simulink model "proj"  (R2015a)
settings: Solver=ode45  StartTime=0.0  StopTime=2.5  RelTol=1e-3
undefined symbols (not defined in the file): D1, Delta, sigbuilder_block
libraries: powerlib x25, powerlib_meascontrol x15, simulink x2, re_lib x1
settings Model: Creator=Lenovo  LastModifiedBy=Lenovo

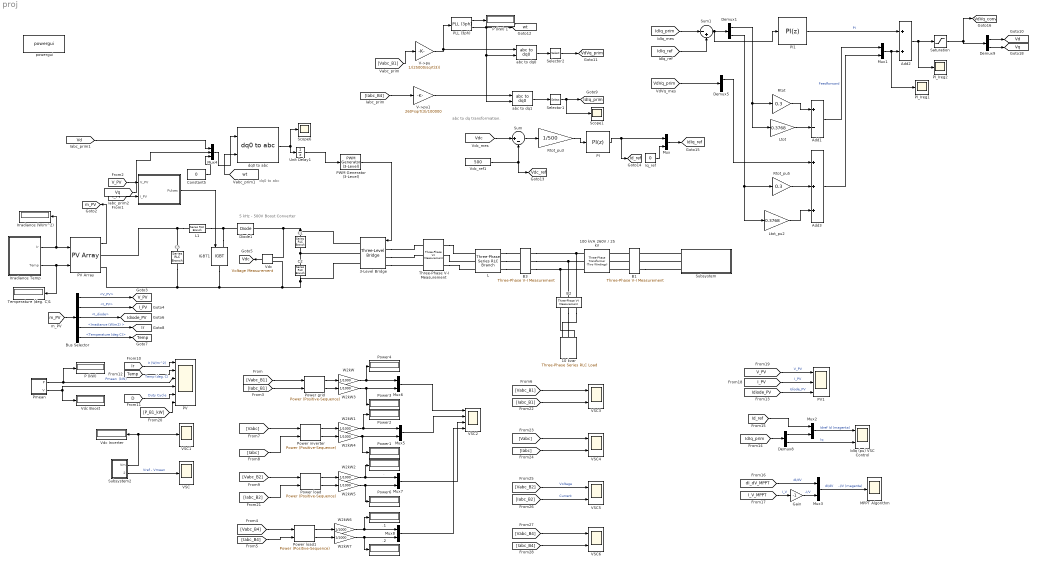
== system proj ==
  note: dq0 to abc
  note: abc to dq transformation.
  note: 5 kHz - 500V
      | Boost Converter
  " " : Subsystem  mask(Boost Control - MPPT){fc=5000, T_MPPT=200e-6, Dinit=0.5}
      mask prompts: fc "PWM switching frequency (Hz)"; T_MPPT "Time window used by MPPT control (s)"; Dinit "Initial value of duty cycle"
  "                                                                                                                                                           ." : Display
      settings: Format=bank  Decimation=2000
  "                                                                                                                                                           .1" : Display
      settings: Format=bank  Decimation=2000
  "                                                                                                                                                           .2" : Display
      settings: Format=bank  Decimation=2000
  10 kvar : powerlib/Elements/Three-Phase Series RLC Load  LConnTagsString=A|B|C  Configuration=Y (grounded)  NominalVoltage=240  NominalFrequency=60  ActivePower=50e3  InductivePower=0  CapacitivePower=0  Measurements=None  LoadType=constant Z
  100 kVA 260V / 25 kV : powerlib/Elements/Three-Phase Transformer (Two Windings)  Winding1Connection=Yg  Winding2Connection=Delta (D1)  CoreType=Three single-phase transformers  SetSaturation=off  Hysteresis=off  DataFile='hysteresis'  SetInitialFlux=off  Measurements=None  UNITS=pu  NominalPower=[100e3 , 60 ]  Winding1=[25000 0.001 0.03]  Winding2=[260 0.001 0.029999]  Rm=500  Lm=500  L0=0.5  Saturation=[0 0;0.0024 1.2;1 1.52]  InitialFluxes=[0.79999 -0.79999 0.7]  MoreParameters=off  BreakLoop=off  DataType=off  TransfoNumber=0
  3-Level Bridge : powerlib/Power Electronics/Three-Level Bridge  Arms=3  SnubberResistance=1e6  SbubberCapacitance=inf  Device=IGBT / Diodes  Ron=0.2e-3  ForwardVoltages="[  0  0 ]"  Measurements=None
  Add1 : Sum  Inputs=+-
  Add2 : Sum
  Add3 : Sum  Inputs=+++
  B1 : powerlib/Measurements/Three-Phase V-I Measurement  VoltageMeasurement=phase-to-ground  SetLabelV=on  LabelV=Vabc_B1  Vpu=off  VpuLL=off  CurrentMeasurement=yes  SetLabelI=on  LabelI=Iabc_B1  Ipu=off  Pbase=100e6  Vbase=500e3  OutputType=Magnitude  PhasorSimulation=off  PSBequivalent=0
  B2 : powerlib/Measurements/Three-Phase V-I Measurement  VoltageMeasurement=phase-to-ground  SetLabelV=on  LabelV=Vabc_B2  Vpu=off  VpuLL=off  CurrentMeasurement=yes  SetLabelI=on  LabelI=Iabc_B2  Ipu=off  Pbase=100e6  Vbase=500e3  OutputType=Magnitude  PhasorSimulation=off  PSBequivalent=0
  B3 : powerlib/Measurements/Three-Phase V-I Measurement  VoltageMeasurement=phase-to-ground  SetLabelV=on  LabelV=Vabc_B4  Vpu=off  VpuLL=off  CurrentMeasurement=yes  SetLabelI=on  LabelI=Iabc_B4  Ipu=off  Pbase=100e6  Vbase=500e3  OutputType=Magnitude  PhasorSimulation=off  PSBequivalent=0
  Bus Selector : BusSelector  OutputSignals=V_PV,I_PV,I_diode,Irradiance (W/m2) ,Temperature (deg C)
  C1 : powerlib/Elements/Series RLC Branch  LConnTagsString=__new0  RConnTagsString=__new0  BranchType=C  Resistance=1.0  Inductance=1.0  SetiL0=off  InitialCurrent=0  Capacitance=12000e-06  Setx0=off  InitialVoltage=0  Measurements=None
  C2 : powerlib/Elements/Series RLC Branch  LConnTagsString=__new0  RConnTagsString=__new0  BranchType=C  Resistance=1.0  Inductance=1.0  SetiL0=off  InitialCurrent=0  Capacitance=12000e-06  Setx0=off  InitialVoltage=0  Measurements=None
  C3 : powerlib/Elements/Series RLC Branch  LConnTagsString=__new0  RConnTagsString=__new0  BranchType=C  Resistance=1.0  Inductance=1.0  SetiL0=off  InitialCurrent=0  Capacitance=100e-6  Setx0=off  InitialVoltage=0  Measurements=Branch voltage
  Constant5 : Constant  Value=0
  Demux{1,5,8..9} (4 alike) : Demux  Outputs=2
  Diode1 : powerlib/Power Electronics/Diode  Ron=1e-4  Lon=0  Vf=0  IC=0  UseSnubber=off  Rs=inf  Cs=inf  Measurements=off
  Gain : Gain  Gain=-1
  IGBT1 : powerlib/Power Electronics/IGBT  Ron=0.001  Lon=0  Vf=0  Tf=0  Tt=0  IC=0  Rs=1e5  Cs=inf  Measurements=off
  IdIq (pu) VSC Control : Scope  NumInputPorts=2
      settings: TimeRange=2  YMin=-5~-5  YMax=5~5  SaveName=ScopeData8  Decimation=100
  Iq_ref : Constant  Value=0
  Irradiance (W/m^2) : Display
      settings: Format=bank  Decimation=1000
  Irradiance Temp : Subsystem  Tag=STV Subsys  LoadFcn=sigbuilder_block('load');  StartFcn=sigbuilder_block('start');  StopFcn=sigbuilder_block('stop');  ClipboardFcn=sigbuilder_block('clipboard');  mask(Sigbuilder block){}
      mask help: Sigbuilder GUI
      mask init:
      | if ~strcmp(get_param(bdroot(gcbh),'SimulationStatus'),'stopped') tuvar = sigbuilder_block('maskInit'); end
      settings: CopyFcn=sigbuilder_block('copy');  DeleteFcn=sigbuilder_block('delete');  ModelCloseFcn=sigbuilder_block('modelClose');  PreSaveFcn=sigbuilder_block('preSave');  PauseFcn=sigbuilder_block('pause')  ContinueFcn=sigbuilder_block('continue')  NameChangeFcn=sigbuilder_block('namechange');  OpenFcn=sigbuilder_block('open',[216.75 153.75 550.5 395.25 ]);  CloseFcn=sigbuilder_block('close');
      mask Display: plot(0,0,100,100,[10,10,40,40,10],[80,20,20,80,80],[40,10],[50,50], [40,27,10],[65,72,56],[40,25,25,10],[28,28,43,43]);
  L : powerlib/Elements/Three-Phase Series RLC Branch  LConnTagsString=A|B|C  RConnTagsString=A|B|C  BranchType=RL  Resistance=0.3  Inductance=1e-3  Capacitance=inf  Measurements=None
  L1 : powerlib/Elements/Series RLC Branch  LConnTagsString=__new0  RConnTagsString=__new0  BranchType=RL  Resistance=0.005  Inductance=5e-3  SetiL0=off  InitialCurrent=0  Capacitance=1e-6  Setx0=off  InitialVoltage=0  Measurements=None
  Ltot : Gain  Gain=0.3768  SaturateOnIntegerOverflow=on  OutDataTypeStr=Inherit: Same as input  ParamDataTypeStr=Inherit: Same as input
  Ltot_pu2 : Gain  Gain=0.3768  SaturateOnIntegerOverflow=on  OutDataTypeStr=Inherit: Same as input  ParamDataTypeStr=Inherit: Same as input
  MPPT Algorithm : Scope
      settings: TimeRange=2  SaveName=ScopeData9  Decimation=100
  Mux{,1..3,5..8} (8 alike) : Mux  Inputs=2
  Mux4 : Mux  Inputs=3
  "P (kW) " : Display
      settings: Format=bank  Decimation=2000
  P (kW) 1 : Display
      settings: Format=bank  Decimation=2000
  PI : simulink/Continuous/PID Controller  Controller=PI  TimeDomain=Discrete-time  SampleTime=1e-06  IntegratorMethod=Trapezoidal  FilterMethod=Forward Euler  Form=Parallel  UseFilter=on  ControllerParametersSource=internal  P=7  I=800  D=0  N=100  InitialConditionSource=internal  InitialConditionForIntegrator=0  InitialConditionForFilter=0  ExternalReset=none  LimitOutput=on  UpperSaturationLimit=1.5  LowerSaturationLimit=-1.5  LinearizeAsGain=off  AntiWindupMode=none  Kb=1  TrackingMode=off  Kt=1  PParamMin=[]  PParamMax=[]  IParamMin=[]  IParamMax=[]  DParamMin=[]  DParamMax=[]  NParamMin=[]  NParamMax=[]  KbParamMin=[]  KbParamMax=[]  KtParamMin=[]  KtParamMax=[]  POutMin=[]  POutMax=[]  IOutMin=[]  IOutMax=[]  DOutMin=[]  DOutMax=[]  NOutMin=[]  NOutMax=[]  KbOutMin=[]  KbOutMax=[]  KtOutMin=[]  KtOutMax=[]  IntegratorOutMin=[]  IntegratorOutMax=[]  FilterOutMin=[]  FilterOutMax=[]  SumOutMin=[]  SumOutMax=[]  SumI1OutMin=[]  SumI1OutMax=[]  SumI2OutMin=[]  SumI2OutMax=[]  SumI3OutMin=[]  SumI3OutMax=[]  SumDOutMin=[]  SumDOutMax=[]  SaturationOutMin=[]  SaturationOutMax=[]  IntegratorContinuousStateAttributes=''  IntegratorStateMustResolveToSignalObject=off  IntegratorRTWStateStorageClass=Auto  FilterContinuousStateAttributes=''  FilterStateMustResolveToSignalObject=off  FilterRTWStateStorageClass=Auto  DifferentiatorICPrevScaledInput=0  DifferentiatorOutMin=[]  DifferentiatorOutMax=[]
  PI1 : simulink/Continuous/PID Controller  Controller=PI  TimeDomain=Discrete-time  SampleTime=1e-06  IntegratorMethod=Forward Euler  FilterMethod=Forward Euler  Form=Parallel  UseFilter=on  ControllerParametersSource=internal  P=0.3  I=20  D=0  N=100  InitialConditionSource=internal  InitialConditionForIntegrator=0  InitialConditionForFilter=0  ExternalReset=none  LimitOutput=on  UpperSaturationLimit=2  LowerSaturationLimit=-2  LinearizeAsGain=off  AntiWindupMode=none  Kb=1  TrackingMode=off  Kt=1  PParamMin=[]  PParamMax=[]  IParamMin=[]  IParamMax=[]  DParamMin=[]  DParamMax=[]  NParamMin=[]  NParamMax=[]  KbParamMin=[]  KbParamMax=[]  KtParamMin=[]  KtParamMax=[]  POutMin=[]  POutMax=[]  IOutMin=[]  IOutMax=[]  DOutMin=[]  DOutMax=[]  NOutMin=[]  NOutMax=[]  KbOutMin=[]  KbOutMax=[]  KtOutMin=[]  KtOutMax=[]  IntegratorOutMin=[]  IntegratorOutMax=[]  FilterOutMin=[]  FilterOutMax=[]  SumOutMin=[]  SumOutMax=[]  SumI1OutMin=[]  SumI1OutMax=[]  SumI2OutMin=[]  SumI2OutMax=[]  SumI3OutMin=[]  SumI3OutMax=[]  SumDOutMin=[]  SumDOutMax=[]  SaturationOutMin=[]  SaturationOutMax=[]  IntegratorContinuousStateAttributes=''  IntegratorStateMustResolveToSignalObject=off  IntegratorRTWStateStorageClass=Auto  FilterContinuousStateAttributes=''  FilterStateMustResolveToSignalObject=off  FilterRTWStateStorageClass=Auto  DifferentiatorICPrevScaledInput=0  DifferentiatorOutMin=[]  DifferentiatorOutMax=[]
  PI_Ireg1 : Scope
      settings: SaveName=ScopeData5
  PI_Ireg2 : Scope
      settings: SaveName=ScopeData13
  PLL (3ph) : powerlib_meascontrol/PLL/PLL (3ph)  Fmin=45  Par_Init="[-0.57  60]"  ParK=[180, 3200, 1]  TcD=1e-4  MaxRateChangeFreq=12  FilterCutOffFreq=25  Ts=1e-06  AGC=on
  PV : Scope  NumInputPorts=6
      settings: TimeRange=2.5  YMin=200~25~0~0~0.44~-5  YMax=1000~50~150~400~0.52~5  SaveName=ScopeData7  Decimation=100
  PV Array : re_lib/Solar/PV Array  Npar=66  Nser=5  PlotType=array @ 1000 W/m2 & specified temperatures  S_vec="[ 1000  250 ]"  Temp_C_vec="[0 25 50  ]"  ModuleName=SunPower SPR-305E-WHT-D  PlotWhenSelected=off  Pm=305.226  Ncell=96  Voc=64.2  Isc=5.96  Vm=54.7  Im=5.58  beta_Voc_pc=-0.27269  alpha_Isc_pc=0.061745  beta_Voc=-0.17507  alpha_Isc=0.00368  IL=6.0092  I0=6.3014e-12  nI=0.94504  Rsh=269.5934  Rs=0.37152  BAL=on  Tc=Tc  Tfilter=5e-5
  PV1 : Scope  NumInputPorts=3
      settings: TimeRange=2  YMin=-5~-5~-5  YMax=5~5~5  SaveName=ScopeData10  Decimation=100
  PWM Generator (3-Level) : powerlib_meascontrol/Pulse & Signal Generators/PWM Generator (3-Level)  ModulatorType=Three-phase bridge (12 pulses)  ModulatorMode=Unsynchronized  nF=27  Fc=33*60  ModulatingSignals=off  m=0.8  Freq=60  Phase=0  Ts=1e-06
  Pmean : Subsystem
  Power grid : powerlib_meascontrol/Measurements/Power (Positive-Sequence)  Freq=60  Vinit=[0, 0]  Iinit=[0, 0]  Ts=1e-06
  Power inverter : powerlib_meascontrol/Measurements/Power (Positive-Sequence)  Freq=60  Vinit=[0, 0]  Iinit=[0, 0]  Ts=1e-06
  Power load : powerlib_meascontrol/Measurements/Power (Positive-Sequence)  Freq=60  Vinit=[0, 0]  Iinit=[0, 0]  Ts=1e-06
  Power load1 : powerlib_meascontrol/Measurements/Power (Positive-Sequence)  Freq=60  Vinit=[0, 0]  Iinit=[0, 0]  Ts=1e-06
  Power{1..4,6} (5 alike) : Display
      settings: Format=bank  Decimation=2000
  Rtot : Gain  Gain=0.3  SaturateOnIntegerOverflow=on  OutDataTypeStr=Inherit: Same as input  ParamDataTypeStr=Inherit: Same as input
  Rtot_pu3 : Gain  Gain=1/500  SaturateOnIntegerOverflow=on  OutDataTypeStr=Inherit: Same as input  ParamDataTypeStr=Inherit: Same as input
  Rtot_pu5 : Gain  Gain=0.3  SaturateOnIntegerOverflow=on  OutDataTypeStr=Inherit: Same as input  ParamDataTypeStr=Inherit: Same as input
  Saturation : Saturate  UpperLimit=2  LowerLimit=-2
  Scope1 : Scope
      settings: YMin=-0.09  YMax=0.06
  Scope6 : Scope
      settings: SaveName=ScopeData14
  Selector1 : Selector  InputPortWidth=3  Indices=[1 2]
  Selector2 : Selector  InputPortWidth=3  Indices=[1 2]
  Subsystem : Subsystem
  Subsystem2 : Subsystem
  Sum : Sum  Inputs=|+-
  Sum1 : Sum  Inputs=|-+
  Temperature (deg. C)1 : Display
      settings: Format=bank  Decimation=1000
  Three-Phase V-I Measurement : powerlib/Measurements/Three-Phase V-I Measurement  VoltageMeasurement=phase-to-ground  SetLabelV=on  LabelV=Vabc  Vpu=off  VpuLL=off  CurrentMeasurement=yes  SetLabelI=on  LabelI=Iabc  Ipu=off  Pbase=100e6  Vbase=500e3  OutputType=Complex  PhasorSimulation=off  PSBequivalent=0
  Unit Delay1 : UnitDelay  SampleTime=1e-06
  V->pu : Gain  Gain=1/(25000/sqrt(3))  SaturateOnIntegerOverflow=on  OutDataTypeStr=Inherit: Same as input  ParamDataTypeStr=Inherit: Same as input
  V->pu1 : Gain  Gain=260*sqrt(3)/100000  SaturateOnIntegerOverflow=on  OutDataTypeStr=Inherit: Same as input  ParamDataTypeStr=Inherit: Same as input
  VSC : Scope
      settings: TimeRange=2.5  SaveName=ScopeData6  Decimation=100
  VSC1 : Scope
      settings: TimeRange=2.5  YMin=499.92  YMax=500.08  SaveName=ScopeData11  Decimation=100
  VSC2 : Scope  NumInputPorts=4
      settings: TimeRange=2.5  YMin=-350~-275~-5~-5  YMax=350~275~5~5  Decimation=100
  VSC{3..6} (4 alike) : Scope  NumInputPorts=2
      VSC3 settings: TimeRange=2.5  YMin=-350~-275  YMax=350~275  SaveName=ScopeData2  Decimation=100
      VSC4 settings: TimeRange=2.5  YMin=-350~-275  YMax=350~275  SaveName=ScopeData3  Decimation=100
      VSC5 settings: TickLabels=on  ShowLegends=on  TimeRange=2.5  YMin=-350~-275  YMax=350~275  SaveName=ScopeData4  Decimation=100
      VSC6 settings: TimeRange=2.5  YMin=-350~-275  YMax=350~275  SaveName=ScopeData12  Decimation=100
  "Vdc " : powerlib/Measurements/Voltage Measurement  Tag=PoWeRsYsTeMmEaSuReMeNt  PhasorSimulation=off  OutputType=Magnitude  PSBequivalent=0
  Vdc Boost : Display
      settings: Format=bank  Decimation=2000
  Vdc Inverter : Display
      settings: Format=bank  Decimation=2000
  Vdc_ref1 : Constant  Value=500
  W2kW{,1..7} (8 alike) : Gain  Gain=1/1000
  abc to dq0 : powerlib_meascontrol/Transformations/abc to dq0  Alignment=90 degrees behind phase A axis
  abc to dq1 : powerlib_meascontrol/Transformations/abc to dq0  Alignment=90 degrees behind phase A axis
  dq0 to abc : powerlib_meascontrol/Transformations/dq0 to abc  Alignment=90 degrees behind phase A axis
  powergui : powerlib/powergui  Priority=1  SimulationMode=Discrete  SolverType=Tustin/Backward Euler (TBE)  SampleTime=1e-06  frequency=60  SPID=off  DisableSnubberDevices=off  DisableRonSwitches=off  DisableVfSwitches=off  SwTol=0  DisplayEquations=off  Interpol=off  methode=off  Ts=0  FunctionMessages=off  echomessages=off  HookPort=off  EnableUseOfTLC=off  x0status=blocks  frequencyindice=0  Pbase=100e6  ErrMax=1e-4  Iterations=50  UnitsV=kV  UnitsW=MW  buscounter=0  RestoreLinks=warning  ResistiveCurrentMeasurement=off  Frange=[0:2:500]  Ylog=off  Xlog=on  ShowGrid=off  save=off  variable=ZData  structure=ScopeData3  ZoomFFT=off  StartTime=0.1  cycles=20  DisplayStyle=1  fundamental=60  FreqAxis=off  MaxFrequency=1000  frequencyindicesteady=1  RmsSteady=1  display=off
  tag scope: I_PV=global, IdIq_prim=global, IdIq_ref=global, Id_ref=global, Idiode_PV=global, Ir=global, Temp=global, V_PV=global, Vd=global, VdVq_conv=global, VdVq_prim=global, Vdc=global, Vdc_ref=global, Vq=global, m_PV=global, wt=global
  wires:
  PV Array/1 -> [m_PV]
  [m_PV] -> Bus Selector/1
  Bus Selector/4 -> [Ir]  "<Irradiance (W/m2) >"
  Bus Selector/5 -> [Temp]  "<Temperature (deg C)>"
  Bus Selector/1 -> [V_PV]  "<V_PV>"
  Bus Selector/2 -> [I_PV]  "<I_PV>"
  Bus Selector/3 -> [Idiode_PV]  "<I_diode>"
  "Vdc "/1 -> [Vdc]
  [I_PV] -> " "/2(I_PV)
  [V_PV] -> " "/1(V_PV)
  [Vabc_B1] -> Power grid/1
  [Iabc_B1] -> Power grid/2
  Power grid/2 -> W2kW3/1
  Power grid/1 -> W2kW/1
  V->pu1/1 -> abc to dq1/1
  V->pu/1 -> PLL (3ph)/1, abc to dq0/1
  abc to dq1/1 -> Selector1/1
  [Vabc_B1] -> V->pu/1
  [Iabc_B4] -> V->pu1/1
  abc to dq0/1 -> Selector2/1
  Selector2/1 -> [VdVq_prim]
  Selector1/1 -> Scope1/1, [IdIq_prim]
  PLL (3ph)/2 -> [wt], abc to dq1/2, abc to dq0/2
  PLL (3ph)/1 -> P (kW) 1/1
  Sum/1 -> Rtot_pu3/1
  [Vdc] -> Sum/1
  Vdc_ref1/1 -> Sum/2, [Vdc_ref]
  Rtot_pu3/1 -> PI/1
  PI/1 -> Mux/1, [Id_ref]
  Iq_ref/1 -> Mux/2
  Mux/1 -> [IdIq_ref]
  Mux1/1 -> PI_Ireg1/1, Add2/2
  PI1/1 -> Add2/1  "PI"
  [IdIq_ref] -> Sum1/2
  [IdIq_prim] -> Sum1/1
  Add2/1 -> PI_Ireg2/1, Saturation/1
  Saturation/1 -> [VdVq_conv], Demux9/1
  [VdVq_prim] -> Demux5/1
  Demux1/1 -> Ltot/1, Rtot/1
  Ltot/1 -> Add1/2
  Demux1/2 -> Rtot_pu5/1, Ltot_pu2/1
  Rtot_pu5/1 -> Add3/2
  Ltot_pu2/1 -> Add3/3
  Add1/1 -> Mux1/1  "Feedforward"
  Add3/1 -> Mux1/2
  Subsystem2/2(VrVm) -> VSC/1  "Vref - Vmean"
  Subsystem2/1(Vm) -> Vdc Inverter/1, VSC1/1
  Pmean/1(P) -> PV/3, "P (kW) "/1  "Pmean  (kW)"
  [D] -> PV/5  "Duty Cycle"
  [Temp] -> PV/2  "Temp (deg. C)"
  [Ir] -> PV/1  "Ir (W/m^2)"
  PWM Generator (3-Level)/1 -> 3-Level Bridge/1
  " "/1(Pulses) -> IGBT1/1
  [I_V_MPPT] -> Gain/1  "I_V"
  [IdIq_prim] -> Demux8/1
  [Id_ref] -> Mux2/1
  Demux8/1 -> Mux2/2
  Mux2/1 -> IdIq (pu) VSC Control/1  "Idref Id (magenta)"
  Demux8/2 -> IdIq (pu) VSC Control/2  "Iq"
  [V_PV] -> PV1/1  "V_PV"
  [I_PV] -> PV1/2  "I_PV"
  [Idiode_PV] -> PV1/3  "Idiode_PV"
  [dI_dV_MPPT] -> Mux3/1  "dI/dV"
  Gain/1 -> Mux3/2  "-I/V"
  Mux3/1 -> MPPT Algorithm/1  "dI/dV     -I/V (magenta)"
  Demux9/1 -> [Vd]
  Demux9/2 -> [Vq]
  [Vq] -> Mux4/2
  [Vd] -> Mux4/1
  Constant5/1 -> Mux4/3
  Mux4/1 -> dq0 to abc/1
  [wt] -> dq0 to abc/2
  dq0 to abc/1 -> Unit Delay1/1, Scope6/1
  Unit Delay1/1 -> PWM Generator (3-Level)/1
  [P_B1_kW] -> PV/6
  [Vabc] -> Power inverter/1
  [Iabc] -> Power inverter/2
  Power inverter/1 -> W2kW1/1
  W2kW1/1 -> Power2/1, Mux5/1
  [Vabc_B2] -> Power load/1
  [Iabc_B2] -> Power load/2
  Power load/1 -> W2kW2/1
  W2kW2/1 -> "                                                                                                                                                           ."/1, Mux7/1
  W2kW3/1 -> Power3/1, Mux6/2
  Power inverter/2 -> W2kW4/1
  W2kW4/1 -> Power1/1, Mux5/2
  [Vabc_B4] -> Power load1/1
  [Iabc_B4] -> Power load1/2
  Sum1/1 -> PI1/1, Demux1/1
  Demux5/1 -> Add3/1
  Rtot/1 -> Add1/1
  Pmean/2(V) -> Vdc Boost/1, PV/4
  W2kW/1 -> Power4/1, Mux6/1
  Power load/2 -> W2kW5/1
  W2kW5/1 -> Power6/1, Mux7/2
  Mux6/1 -> VSC2/1
  Mux5/1 -> VSC2/2
  Mux7/1 -> VSC2/3
  Power load1/1 -> W2kW6/1
  Power load1/2 -> W2kW7/1
  W2kW6/1 -> "                                                                                                                                                           .1"/1, Mux8/1
  W2kW7/1 -> "                                                                                                                                                           .2"/1, Mux8/2
  Mux8/1 -> VSC2/4
  [Vabc_B1] -> VSC3/1
  [Iabc_B1] -> VSC3/2
  [Vabc] -> VSC4/1
  [Iabc] -> VSC4/2
  [Vabc_B2] -> VSC5/1  "Voltage"
  [Iabc_B2] -> VSC5/2  "Current"
  [Vabc_B4] -> VSC6/1
  [Iabc_B4] -> VSC6/2
  Irradiance Temp/1(Ir) -> PV Array/1, Irradiance (W/m^2)/1
  Irradiance Temp/2(Temp) -> PV Array/2, Temperature (deg. C)1/1
  connections:
  Diode1/RConn1 -- "Vdc "/LConn1 -- 3-Level Bridge/RConn1 -- C1/LConn1
  IGBT1/LConn1 -- L1/RConn1 -- Diode1/LConn1
  IGBT1/RConn1 -- PV Array/RConn2 -- C3/RConn1 -- 3-Level Bridge/RConn3 -- C2/RConn1 -- "Vdc "/LConn2
  C2/LConn1 -- 3-Level Bridge/RConn2 -- C1/RConn1
  L1/LConn1 -- PV Array/RConn1 -- C3/LConn1
  B2/LConn2 -- B3/RConn2 -- 100 kVA 260V / 25 kV/RConn2
  3-Level Bridge/LConn1 -- Three-Phase V-I Measurement/LConn1
  3-Level Bridge/LConn2 -- Three-Phase V-I Measurement/LConn2
  3-Level Bridge/LConn3 -- Three-Phase V-I Measurement/LConn3
  Three-Phase V-I Measurement/RConn1 -- L/LConn1
  Three-Phase V-I Measurement/RConn2 -- L/LConn2
  Three-Phase V-I Measurement/RConn3 -- L/LConn3
  B1/LConn1 -- 100 kVA 260V / 25 kV/LConn1
  B1/LConn2 -- 100 kVA 260V / 25 kV/LConn2
  B1/LConn3 -- 100 kVA 260V / 25 kV/LConn3
  B2/LConn1 -- 100 kVA 260V / 25 kV/RConn1 -- B3/RConn1
  B2/LConn3 -- 100 kVA 260V / 25 kV/RConn3 -- B3/RConn3
  Subsystem/LConn1 -- B1/RConn1
  Subsystem/LConn2 -- B1/RConn2
  B1/RConn3 -- Subsystem/LConn3
  B2/RConn1 -- 10 kvar/LConn1
  B2/RConn2 -- 10 kvar/LConn2
  10 kvar/LConn3 -- B2/RConn3
  L/RConn1 -- B3/LConn1
  L/RConn2 -- B3/LConn2
  L/RConn3 -- B3/LConn3

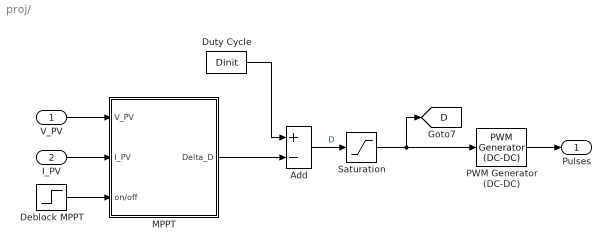
== system proj/  ==
  V_PV : Inport
  I_PV : Inport  Port=2
  Add : Sum  Inputs=+-
  Deblock MPPT : Step  Time=0.1  SampleTime=0
  Duty Cycle : Constant  Value=Dinit
  MPPT : Subsystem
  PWM Generator (DC-DC) : powerlib_meascontrol/Pulse & Signal Generators/PWM Generator (DC-DC)  Fsw=fc  Ts=1e-06
  Saturation : Saturate  UpperLimit=1  LowerLimit=0
  Pulses : Outport
  tag scope: D=global
  wires:
  V_PV/1 -> MPPT/1(V_PV)
  I_PV/1 -> MPPT/2(I_PV)
  PWM Generator (DC-DC)/1 -> Pulses/1
  Deblock MPPT/1 -> MPPT/3(on/off)
  Saturation/1 -> PWM Generator (DC-DC)/1, [D]
  Add/1 -> Saturation/1  "D"
  MPPT/1(Delta_D) -> Add/2
  Duty Cycle/1 -> Add/1

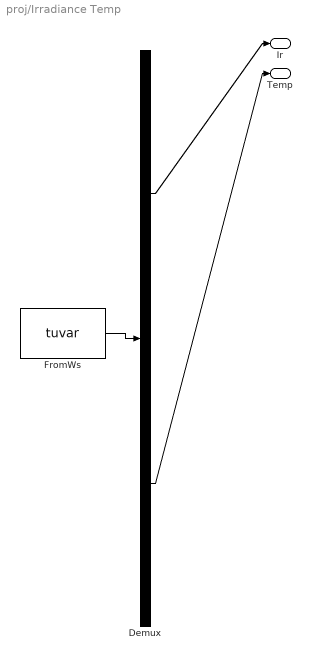
== system proj/Irradiance Temp ==
  Demux : Demux  Tag=STV Demux  Outputs=2
  FromWs : FromWorkspace  Tag=STV FromWs  VariableName=tuvar  SampleTime=0
      SigBuilderData=|
      | common.afterFinalStr = 'Extrapolate'
      | common.sampleTime = '0'
      | dataSet(1).timeRange = [0 1]
      | dataSet(1).name = 'Constant Irradiance'
      | dataSet(2).timeRange = [0 1]
      | dataSet(2).name = 'Step Irradiance'
      | dataSet(3).timeRange = [0 3]
      | dataSet(3).name = 'Ramp-up/down Irradiance'
      | sbobj.Groups(1).Name = 'Constant Irradiance'
      | sbobj.Groups(1).Signals(1).Name = 'Ir'
      | sbobj.Groups(1).Signals(1).XData = [0 1]
      | sbobj.Groups(1).Signals(1).YData = [1000 1000]
      | sbobj.Groups(1).Signals(2).Name = 'Temp'
      | sbobj.Groups(1).Signals(2).XData = [0 1 1 2]
      | sbobj.Groups(1).Signals(2).YData = [0 0 1 1]
      | sbobj.Groups(1).TimeRange = [0 1]
      | sbobj.Groups(2).Name = 'Step Irradiance'
      | sbobj.Groups(2).Signals(1).Name = 'Ir'
      | sbobj.Groups(2).Signals(1).XData = [0 0.252 0.252 1]
      | sbobj.Groups(2).Signals(1).YData = [600 600 1000 1000]
      | sbobj.Groups(2).Signals(2).Name = 'Temp'
      | sbobj.Groups(2).Signals(2).XData = [0 1 1 2]
      | sbobj.Groups(2).Signals(2).YData = [0 0 1 1]
      | sbobj.Groups(2).TimeRange = [0 1]
      | sbobj.Groups(3).Name = 'Ramp-up/down Irradiance'
      | sbobj.Groups(3).Signals(1).Name = 'Ir'
      | sbobj.Groups(3).Signals(1).XData = [0 0.6 1.1 1.2 1.7 3]
      | sbobj.Groups(3).Signals(1).YData = [1000 1000 250 250 1000 1000]
      | sbobj.Groups(3).Signals(2).Name = 'Temp'
      | sbobj.Groups(3).Signals(2).XData = [0 2 2.1 3]
      | sbobj.Groups(3).Signals(2).YData = [25 25 25 25]
      | sbobj.Groups(3).TimeRange = [0 3]
  Ir : Outport  Tag=STV Outport
  Temp : Outport  Tag=STV Outport  Port=2
  wires:
  Demux/1 -> Ir/1
  FromWs/1 -> Demux/1
  Demux/2 -> Temp/1

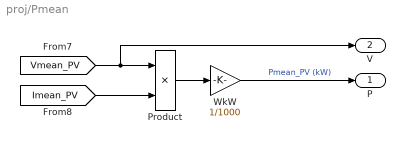
== system proj/Pmean ==
  Product : Product  RndMeth=Zero
  WkW : Gain  Gain=1/1000
  P : Outport
  V : Outport  Port=2
  wires:
  [Vmean_PV] -> Product/1, V/1
  Product/1 -> WkW/1
  [Imean_PV] -> Product/2
  WkW/1 -> P/1  "Pmean_PV (kW)"

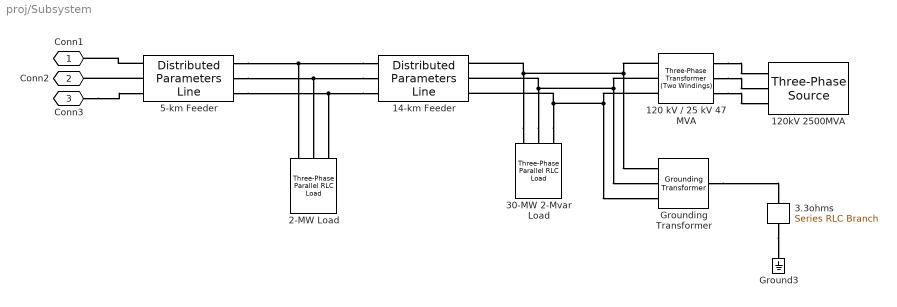
== system proj/Subsystem ==
  120 kV / 25 kV 47 MVA : powerlib/Elements/Three-Phase Transformer (Two Windings)  Winding1Connection=Yg  Winding2Connection=Delta (D1)  CoreType=Three single-phase transformers  SetSaturation=off  Hysteresis=off  DataFile='basic_model'  SetInitialFlux=off  Measurements=None  UNITS=pu  NominalPower=[47e6 60 ]  Winding1="[ 120e3  0.08/30   0.08 ]"  Winding2="[ 25e3  0.08/30  0.08]"  Rm=500  Lm=500  L0=0.5  Saturation="[ 0,0  ;  0.005,1.2  ;  1.0,1.4 ]"  InitialFluxes=[ 0.8 , -0.8 , 0.7 ]  MoreParameters=off  BreakLoop=off  DataType=off  TransfoNumber=0
  120kV 2500MVA : powerlib/Electrical Sources/Three-Phase Source  Voltage=120e3  PhaseAngle=0  Frequency=60  InternalConnection=Yg  SpecifyImpedance=on  Resistance=0.8929  Inductance=16.58e-3  ShortCircuitLevel=2500e6  BaseVoltage=120e3  XRratio=7  BusType=swing  Pref=0  Qref=0  Qmin=-inf  Qmax=inf
  14-km Feeder : powerlib/Elements/Distributed Parameters Line  Phases=3  Frequency=60  Resistance=[0.1153 0.413]  Inductance=[1.05e-3 3.32e-3]  Capacitance=[11.33e-009 5.01e-009]  Length=14  x1=[-5.8e-05 -1.33022205256293e-09 0 0;-5.7e-05 -1.33026516254751e-09 0 0;-5.6e-05 -1.33030808347174e-09 0 0;-5.5e-05 -1.33035081532953e-09 0 0;-5.4e-05 -1.3303933581148e-09 0 0;-5.3e-05 -1.3304357118215e-09 0 0;-5.2e-05 -1.33047787644361e-09 0 0;-5.1e-05 -1.33051985197515e-09 0 0;-5e-05 -1.33056163841014e-09 0 0;-4.9e-05 -1.33060323574265e-09 -3805.56439501913 -24049.8385262992;-4.8e-05 -1.33064464396677e-09 -3796.497549282 -24051.2714812336;-4.7e-05 -1.33068586307661e-09 -3787.43016397789 -24052.7010179458;-4.6e-05 -1.3307268930663e-09 -3778.36224039549 -24054.1271362329;-4.5e-05 -1.33076773393003e-09 -3769.29377982355 -24055.5498358921;-4.4e-05 -1.33080838566199e-09 -3760.22478355091 -24056.9691167211;-4.3e-05 -1.3308488482564e-09 -3751.15525286646 -24058.3849785183;-4.2e-05 -1.3308891217075e-09 -3742.0851890592 -24059.7974210825;-4.1e-05 -1.33092920600958e-09 -3733.01459341817 -24061.2064442128;-4e-05 -1.33096910115694e-09 -3723.94346723252 -24062.6120477092;-3.9e-05 -1.3310088071439e-09 -3714.87181179146 -24064.0142313717;-3.8e-05 -1.33104832396483e-09 -3705.79962838425 -24065.4129950011;-3.7e-05 -1.33108765161411e-09 -3696.72691830028 -24066.8083383987;-3.6e-05 -1.33112679008615e-09 -3687.65368282897 -24068.200261366;-3.5e-05 -1.33116573937538e-09 -3678.57992325983 -24069.5887637054;-3.4e-05 -1.33120449947628e-09 -3669.50564088244 -24070.9738452194;-3.3e-05 -1.33124307038332e-09 -3660.43083698647 -24072.3555057111;-3.2e-05 -1.33128145209104e-09 -3651.35551286164 -24073.7337449843;-3.1e-05 -1.33131964459398e-09 -3642.27966979776 -24075.1085628431;-3e-05 -1.3313576478867e-09 -3633.20330908471 -24076.479959092;-2.9e-05 -1.33139546196381e-09 -3624.12643201244 -24077.8479335362;-2.8e-05 -1.33143308681993e-09 -3615.04903987099 -24079.2124859811;-2.7e-05 -1.33147052244971e-09 -3605.97113395044 -24080.573616233;-2.6e-05 -1.33150776884784e-09 -3596.89271554098 -24081.9313240984;-2.5e-05 -1.33154482600903e-09 -3587.81378593284 -24083.2856093842;-2.4e-05 -1.33158169392799e-09 -3578.73434641635 -24084.6364718981;-2.3e-05 -1.33161837259951e-09 -3569.6543982819 -24085.9839114479;-2.2e-05 -1.33165486201835e-09 -3560.57394281995 -24087.3279278423;-2.1e-05 -1.33169116217934e-09 -3551.49298132103 -24088.6685208903;-2e-05 -1.33172727307731e-09 -3542.41151507576 -24090.0056904012;-1.9e-05 -1.33176319470715e-09 -3533.32954537481 -24091.339436185;-1.8e-05 -1.33179892706373e-09 -3524.24707350893 -24092.6697580523;-1.7e-05 -1.33183447014198e-09 -3515.16410076895 -24093.9966558138;-1.6e-05 -1.33186982393685e-09 -3506.08062844575 -24095.3201292811;-1.5e-05 -1.33190498844331e-09 -3496.99665783031 -24096.6401782661;-1.4e-05 -1.33193996365638e-09 -3487.91219021365 -24097.956802581;-1.3e-05 -1.33197474957107e-09 -3478.82722688688 -24099.2700020389;-1.2e-05 -1.33200934618244e-09 -3469.74176914118 -24100.5797764531;-1.1e-05 -1.33204375348558e-09 -3460.65581826779 -24101.8861256374;-1e-05 -1.3320779714756e-09 -3451.56937555803 -24103.1890494061;-9e-06 -1.33211200014762e-09 -3442.48244230329 -24104.4885475742;-8e-06 -1.33214583949683e-09 -3433.39501979502 -24105.7846199569;-7e-06 -1.3321794895184e-09 -3424.30710932475 -24107.0772663699;-6e-06 -1.33221295020755e-09 -3415.21871218407 -24108.3664866297;-5e-06 -1.33224622155954e-09 -3406.12982966465 -24109.6522805529;-4e-06 -1.33227930356962e-09 -3397.04046305821 -24110.9346479569;-3e-06 -1.33231219623311e-09 -3387.95061365656 -24112.2135886593;-2e-06 -1.33234489954532e-09 -3378.86028275158 -24113.4891024784;-1e-06 -1.3323774135016e-09 -3369.76947163519 -24114.761189233]  x2=[-5.8e-05 -1.51928848261934e-09 0 0;-5.7e-05 -1.51928718215419e-09 0 0;-5.6e-05 -1.51928566576445e-09 0 0;-5.5e-05 -1.51928393345033e-09 0 0;-5.4e-05 -1.51928198521209e-09 0 0;-5.3e-05 -1.51927982104999e-09 0 0;-5.2e-05 -1.51927744096435e-09 0 0;-5.1e-05 -1.5192748449555e-09 0 0;-5e-05 -1.51927203302381e-09 0 0;-4.9e-05 -1.51926900516969e-09 -3383.9503694369 -24241.1103133339;-4.8e-05 -1.51926576139356e-09 -3374.81144589693 -24242.384309937;-4.7e-05 -1.51926230169588e-09 -3365.67204272099 -24243.6548611566;-4.6e-05 -1.51925862607714e-09 -3356.53216120799 -24244.9219668122;-4.5e-05 -1.51925473453787e-09 -3347.39180265692 -24246.1856267236;-4.4e-05 -1.51925062707863e-09 -3338.25096836682 -24247.4458407114;-4.3e-05 -1.51924630369998e-09 -3329.1096596368 -24248.7026085964;-4.2e-05 -1.51924176440256e-09 -3319.96787776606 -24249.9559301999;-4.1e-05 -1.519237009187e-09 -3310.82562405385 -24251.2058053439;-4e-05 -1.51923203805397e-09 -3301.68289979947 -24252.4522338506;-3.9e-05 -1.5192268510042e-09 -3292.53970630233 -24253.6952155431;-3.8e-05 -1.5192214480384e-09 -3283.39604486186 -24254.9347502445;-3.7e-05 -1.51921582915736e-09 -3274.25191677759 -24256.1708377788;-3.6e-05 -1.51920999436187e-09 -3265.10732334909 -24257.4034779703;-3.5e-05 -1.51920394365276e-09 -3255.96226587604 -24258.6326706438;-3.4e-05 -1.51919767703088e-09 -3246.81674565813 -24259.8584156245;-3.3e-05 -1.51919119449714e-09 -3237.67076399515 -24261.0807127384;-3.2e-05 -1.51918449605244e-09 -3228.52432218695 -24262.2995618116;-3.1e-05 -1.51917758169775e-09 -3219.37742153344 -24263.5149626709;-3e-05 -1.51917045143404e-09 -3210.2300633346 -24264.7269151437;-2.9e-05 -1.51916310526234e-09 -3201.08224889048 -24265.9354190576;-2.8e-05 -1.51915554318367e-09 -3191.93397950118 -24267.1404742409;-2.7e-05 -1.51914776519912e-09 -3182.78525646687 -24268.3420805223;-2.6e-05 -1.5191397713098e-09 -3173.6360810878 -24269.5402377312;-2.5e-05 -1.51913156151684e-09 -3164.48645466427 -24270.7349456971;-2.4e-05 -1.5191231358214e-09 -3155.33637849663 -24271.9262042503;-2.3e-05 -1.51911449422468e-09 -3146.18585388533 -24273.1140132214;-2.2e-05 -1.51910563672792e-09 -3137.03488213085 -24274.2983724418;-2.1e-05 -1.51909656333236e-09 -3127.88346453376 -24275.4792817429;-2e-05 -1.51908727403931e-09 -3118.73160239466 -24276.6567409571;-1.9e-05 -1.51907776885007e-09 -3109.57929701426 -24277.830749917;-1.8e-05 -1.51906804776601e-09 -3100.42654969328 -24279.0013084557;-1.7e-05 -1.5190581107885e-09 -3091.27336173255 -24280.1684164068;-1.6e-05 -1.51904795791896e-09 -3082.11973443294 -24281.3320736045;-1.5e-05 -1.51903758915882e-09 -3072.96566909537 -24282.4922798834;-1.4e-05 -1.51902700450956e-09 -3063.81116702085 -24283.6490350786;-1.3e-05 -1.51901620397269e-09 -3054.65622951043 -24284.8023390257;-1.2e-05 -1.51900518754974e-09 -3045.50085786524 -24285.9521915608;-1.1e-05 -1.51899395524228e-09 -3036.34505338646 -24287.0985925205;-1e-05 -1.5189825070519e-09 -3027.18881737533 -24288.2415417418;-9e-06 -1.51897084298023e-09 -3018.03215113316 -24289.3810390623;-8e-06 -1.51895896302893e-09 -3008.87505596131 -24290.5170843201;-7e-06 -1.51894686719968e-09 -2999.71753316121 -24291.6496773537;-6e-06 -1.51893455549421e-09 -2990.55958403436 -24292.7788180022;-5e-06 -1.51892202791426e-09 -2981.40120988229 -24293.904506105;-4e-06 -1.51890928446162e-09 -2972.24241200662 -24295.0267415021;-3e-06 -1.5188963251381e-09 -2963.08319170902 -24296.1455240342;-2e-06 -1.51888314994553e-09 -2953.92355029121 -24297.2608535421;-1e-06 -1.51886975888579e-09 -2944.76348905499 -24298.3727298674]  x3=[-5.8e-05 -1.05183303206471e-11 0 0;-5.7e-05 -1.05211088090771e-11 0 0;-5.6e-05 -1.05238858022228e-11 0 0;-5.5e-05 -1.05266612996898e-11 0 0;-5.4e-05 -1.05294353010833e-11 0 0;-5.3e-05 -1.05322078060093e-11 0 0;-5.2e-05 -1.05349788140737e-11 0 0;-5.1e-05 -1.05377483248827e-11 0 0;-5e-05 -1.05405163380426e-11 0 0;-4.9e-05 -1.054328285316e-11 -24.5285615763521 -157.764393315577;-4.8e-05 -1.05460478698419e-11 -24.4690840596485 -157.773629154301;-4.7e-05 -1.05488113876951e-11 -24.4096030653423 -157.782842569873;-4.6e-05 -1.0551573406327e-11 -24.3501186018872 -157.792033560985;-4.5e-05 -1.0554333925345e-11 -24.2906306777372 -157.80120212633;-4.4e-05 -1.05570929443567e-11 -24.2311393013468 -157.810348264604;-4.3e-05 -1.05598504629701e-11 -24.1716444811711 -157.819471974509;-4.2e-05 -1.05626064807933e-11 -24.1121462256657 -157.828573254747;-4.1e-05 -1.05653609974345e-11 -24.0526445432866 -157.837652104025;-4e-05 -1.05681140125023e-11 -23.9931394424902 -157.846708521053;-3.9e-05 -1.05708655256054e-11 -23.9336309317337 -157.855742504543;-3.8e-05 -1.05736155363527e-11 -23.8741190194744 -157.864754053212;-3.7e-05 -1.05763640443535e-11 -23.8146037141704 -157.873743165778;-3.6e-05 -1.05791110492171e-11 -23.7550850242801 -157.882709840965;-3.5e-05 -1.05818565505531e-11 -23.6955629582625 -157.891654077497;-3.4e-05 -1.05846005479712e-11 -23.6360375245769 -157.900575874104;-3.3e-05 -1.05873430410816e-11 -23.5765087316832 -157.909475229518;-3.2e-05 -1.05900840294944e-11 -23.5169765880419 -157.918352142474;-3.1e-05 -1.05928235128201e-11 -23.4574411021137 -157.92720661171;-3e-05 -1.05955614906693e-11 -23.3979022823599 -157.936038635968;-2.9e-05 -1.05982979626529e-11 -23.3383601372425 -157.944848213993;-2.8e-05 -1.06010329283821e-11 -23.2788146752236 -157.953635344533;-2.7e-05 -1.0603766387468e-11 -23.219265904766 -157.962400026338;-2.6e-05 -1.06064983395223e-11 -23.1597138343329 -157.971142258163;-2.5e-05 -1.06092287841566e-11 -23.1001584723879 -157.979862038766;-2.4e-05 -1.06119577209828e-11 -23.0405998273952 -157.988559366907;-2.3e-05 -1.06146851496133e-11 -22.9810379078195 -157.997234241351;-2.2e-05 -1.06174110696602e-11 -22.9214727221257 -158.005886660864;-2.1e-05 -1.06201354807362e-11 -22.8619042787795 -158.014516624217;-2e-05 -1.06228583824542e-11 -22.8023325862469 -158.023124130183;-1.9e-05 -1.0625579774427e-11 -22.7427576529942 -158.031709177539;-1.8e-05 -1.0628299656268e-11 -22.6831794874885 -158.040271765064;-1.7e-05 -1.06310180275906e-11 -22.6235980981971 -158.048811891543;-1.6e-05 -1.06337348880085e-11 -22.5640134935878 -158.05732955576;-1.5e-05 -1.06364502371354e-11 -22.5044256821291 -158.065824756506;-1.4e-05 -1.06391640745856e-11 -22.4448346722895 -158.074297492573;-1.3e-05 -1.06418763999733e-11 -22.3852404725384 -158.082747762757;-1.2e-05 -1.0644587212913e-11 -22.3256430913454 -158.091175565858;-1.1e-05 -1.06472965130195e-11 -22.2660425371806 -158.099580900676;-1e-05 -1.06500042999077e-11 -22.2064388185146 -158.107963766018;-9e-06 -1.06527105731928e-11 -22.1468319438184 -158.116324160693;-8e-06 -1.06554153324901e-11 -22.0872219215635 -158.124662083511;-7e-06 -1.06581185774153e-11 -22.0276087602217 -158.132977533289;-6e-06 -1.06608203075841e-11 -21.9679924682655 -158.141270508843;-5e-06 -1.06635205226126e-11 -21.9083730541677 -158.149541008997;-4e-06 -1.06662192221171e-11 -21.8487505264014 -158.157789032574;-3e-06 -1.06689164057139e-11 -21.7891248934404 -158.166014578401;-2e-06 -1.06716120730197e-11 -21.7294961637589 -158.174217645311;-1e-06 -1.06743062236515e-11 -21.6698643458313 -158.182398232137]  x4=[-5.8e-05 7.68573184031791e-12 0 0;-5.7e-05 7.68885282824083e-12 0 0;-5.6e-05 7.69197272340629e-12 0 0;-5.5e-05 7.69509152537087e-12 0 0;-5.4e-05 7.69820923369134e-12 0 0;-5.3e-05 7.7013258479246e-12 0 0;-5.2e-05 7.7044413676277e-12 0 0;-5.1e-05 7.70755579235786e-12 0 0;-5e-05 7.71066912167244e-12 0 0;-4.9e-05 7.71378135512899e-12 -0.434535278580712 -0.0219978394147175;-4.8e-05 7.71689249228518e-12 -0.434526954712246 -0.0221616537883163;-4.7e-05 7.72000253269884e-12 -0.43451856908781 -0.0223254650122499;-4.6e-05 7.72311147592797e-12 -0.434510121708595 -0.022489273063237;-4.5e-05 7.72621932153073e-12 -0.434501612575801 -0.0226530779179968;-4.4e-05 7.7293260690654e-12 -0.434493041690637 -0.022816879553249;-4.3e-05 7.73243171809047e-12 -0.434484409054323 -0.0229806779457138;-4.2e-05 7.73553626816455e-12 -0.434475714668084 -0.0231444730721118;-4.1e-05 7.7386397188464e-12 -0.434466958533156 -0.023308264909164;-4e-05 7.74174206969497e-12 -0.434458140650785 -0.0234720534335919;-3.9e-05 7.74484332026934e-12 -0.434449261022222 -0.0236358386221176;-3.8e-05 7.74794347012874e-12 -0.434440319648731 -0.0237996204514635;-3.7e-05 7.75104251883259e-12 -0.434431316531581 -0.0239633988983525;-3.6e-05 7.75414046594043e-12 -0.434422251672053 -0.0241271739395081;-3.5e-05 7.75723731101199e-12 -0.434413125071435 -0.0242909455516543;-3.4e-05 7.76033305360712e-12 -0.434403936731023 -0.0244547137115153;-3.3e-05 7.76342769328586e-12 -0.434394686652124 -0.0246184783958162;-3.2e-05 7.76652122960838e-12 -0.434385374836052 -0.0247822395812822;-3.1e-05 7.76961366213503e-12 -0.434376001284131 -0.0249459972446393;-3e-05 7.7727049904263e-12 -0.434366565997692 -0.0251097513626139;-2.9e-05 7.77579521404285e-12 -0.434357068978078 -0.0252735019119328;-2.8e-05 7.77888433254549e-12 -0.434347510226637 -0.0254372488693234;-2.7e-05 7.78197234549518e-12 -0.434337889744729 -0.0256009922115137;-2.6e-05 7.78505925245305e-12 -0.434328207533719 -0.025764731915232;-2.5e-05 7.78814505298038e-12 -0.434318463594986 -0.0259284679572074;-2.4e-05 7.7912297466386e-12 -0.434308657929912 -0.0260922003141692;-2.3e-05 7.79431333298933e-12 -0.434298790539892 -0.0262559289628474;-2.2e-05 7.7973958115943e-12 -0.434288861426329 -0.0264196538799725;-2.1e-05 7.80047718201543e-12 -0.434278870590633 -0.0265833750422757;-2e-05 7.80355744381479e-12 -0.434268818034225 -0.0267470924264884;-1.9e-05 7.80663659655461e-12 -0.434258703758532 -0.0269108060093428;-1.8e-05 7.80971463979727e-12 -0.434248527764993 -0.0270745157675714;-1.7e-05 7.8127915731053e-12 -0.434238290055054 -0.0272382216779076;-1.6e-05 7.81586739604141e-12 -0.434227990630169 -0.027401923717085;-1.5e-05 7.81894210816846e-12 -0.434217629491803 -0.027565621861838;-1.4e-05 7.82201570904946e-12 -0.434207206641428 -0.0277293160889013;-1.3e-05 7.82508819824758e-12 -0.434196722080525 -0.0278930063750104;-1.2e-05 7.82815957532616e-12 -0.434186175810585 -0.0280566926969012;-1.1e-05 7.83122983984868e-12 -0.434175567833106 -0.0282203750313103;-1e-05 7.83429899137879e-12 -0.434164898149596 -0.0283840533549747;-9e-06 7.8373670294803e-12 -0.434154166761572 -0.0285477276446321;-8e-06 7.84043395371717e-12 -0.434143373670558 -0.0287113978770208;-7e-06 7.84349976365351e-12 -0.434132518878088 -0.0288750640288795;-6e-06 7.84656445885362e-12 -0.434121602385706 -0.0290387260769477;-5e-06 7.84962803888192e-12 -0.434110624194962 -0.0292023839979653;-4e-06 7.85269050330302e-12 -0.434099584307417 -0.0293660377686728;-3e-06 7.85575185168167e-12 -0.43408848272464 -0.0295296873658115;-2e-06 7.85881208358279e-12 -0.434077319448209 -0.029693332766123;-1e-06 7.86187119857144e-12 -0.43406609447971 -0.0298569739463497]  x5=5.70973484498186e-05  V1=ones(3,3)  V2=ones(3,3)  I1=ones(3,3)  I2=ones(3,3)  nHarmo=1  Measurements=None
  2-MW Load : powerlib/Elements/Three-Phase Parallel RLC Load  LConnTagsString=A|B|C  Configuration=Y (grounded)  NominalVoltage=25e3  NominalFrequency=60  ActivePower=2e6  InductivePower=0  CapacitivePower=0  Measurements=None  LoadType=constant Z
  "3.3ohms " : powerlib/Elements/Series RLC Branch  LConnTagsString=__new0  RConnTagsString=__new0  BranchType=R  Resistance=3.3  Inductance=[]  SetiL0=off  InitialCurrent=0  Capacitance=[]  Setx0=off  InitialVoltage=0  Measurements=None
  30-MW 2-Mvar Load : powerlib/Elements/Three-Phase Parallel RLC Load  LConnTagsString=A|B|C  Configuration=Y (grounded)  NominalVoltage=25e3  NominalFrequency=60  ActivePower=30e6  InductivePower=2e6  CapacitivePower=0  Measurements=None  LoadType=constant Z
  5-km Feeder : powerlib/Elements/Distributed Parameters Line  Phases=3  Frequency=60  Resistance=[0.1153 0.413]  Inductance=[1.05e-3 3.32e-3]  Capacitance=[11.33e-009 5.01e-009]  Length=5  x1=[-2.1e-05 -1.28776317603057e-09 -3555.92780838445 -24087.0241198561;-2e-05 -1.28781218846346e-09 -3546.8469617486 -24088.3629613743;-1.9e-05 -1.28786101786951e-09 -3537.7656110267 -24089.6983793988;-1.8e-05 -1.28790966424179e-09 -3528.68375750941 -24091.03037374;-1.7e-05 -1.28795812757339e-09 -3519.60140248746 -24092.3589442084;-1.6e-05 -1.28800640785741e-09 -3510.51854725166 -24093.6840906154;-1.5e-05 -1.288054505087e-09 -3501.43519309288 -24095.0058127726;-1.4e-05 -1.28810241925532e-09 -3492.35134130208 -24096.324110492;-1.3e-05 -1.28815015035555e-09 -3483.26699317026 -24097.6389835864;-1.2e-05 -1.28819769838092e-09 -3474.18214998852 -24098.9504318689;-1.1e-05 -1.28824506332467e-09 -3465.09681304802 -24100.2584551531;-1e-05 -1.28829224518007e-09 -3456.01098363998 -24101.563053253;-9e-06 -1.28833924394041e-09 -3446.92466305571 -24102.8642259834;-8e-06 -1.28838605959901e-09 -3437.83785258657 -24104.1619731592;-7e-06 -1.28843269214921e-09 -3428.750553524 -24105.4562945961;-6e-06 -1.2884791415844e-09 -3419.66276715951 -24106.74719011;-5e-06 -1.28852540789796e-09 -3410.57449478468 -24108.0346595175;-4e-06 -1.28857149108333e-09 -3401.48573769114 -24109.3187026356;-3e-06 -1.28861739113395e-09 -3392.39649717063 -24110.5993192819;-2e-06 -1.28866310804331e-09 -3383.30677451492 -24111.8765092743;-1e-06 -1.28870864180489e-09 -3374.21657101586 -24113.1502724313]  x2=[-2.1e-05 -1.33169116217934e-09 -3551.49298132103 -24088.6685208903;-2e-05 -1.33172727307731e-09 -3542.41151507576 -24090.0056904012;-1.9e-05 -1.33176319470715e-09 -3533.32954537481 -24091.339436185;-1.8e-05 -1.33179892706373e-09 -3524.24707350893 -24092.6697580523;-1.7e-05 -1.33183447014198e-09 -3515.16410076895 -24093.9966558138;-1.6e-05 -1.33186982393685e-09 -3506.08062844575 -24095.3201292811;-1.5e-05 -1.33190498844331e-09 -3496.99665783031 -24096.6401782661;-1.4e-05 -1.33193996365638e-09 -3487.91219021365 -24097.956802581;-1.3e-05 -1.33197474957107e-09 -3478.82722688688 -24099.2700020389;-1.2e-05 -1.33200934618244e-09 -3469.74176914118 -24100.5797764531;-1.1e-05 -1.33204375348558e-09 -3460.65581826779 -24101.8861256374;-1e-05 -1.3320779714756e-09 -3451.56937555803 -24103.1890494061;-9e-06 -1.33211200014762e-09 -3442.48244230329 -24104.4885475742;-8e-06 -1.33214583949683e-09 -3433.39501979502 -24105.7846199569;-7e-06 -1.3321794895184e-09 -3424.30710932475 -24107.0772663699;-6e-06 -1.33221295020755e-09 -3415.21871218407 -24108.3664866297;-5e-06 -1.33224622155954e-09 -3406.12982966465 -24109.6522805529;-4e-06 -1.33227930356962e-09 -3397.04046305821 -24110.9346479569;-3e-06 -1.33231219623311e-09 -3387.95061365656 -24112.2135886593;-2e-06 -1.33234489954532e-09 -3378.86028275158 -24113.4891024784;-1e-06 -1.3323774135016e-09 -3369.76947163519 -24114.761189233]  x3=[-2.1e-05 -9.5237296543593e-12 -12.0852906194321 -81.2593037747329;-2e-05 -9.52643076730205e-12 -12.0546557255502 -81.2638540474725;-1.9e-05 -9.52913052632652e-12 -12.0240191184328 -81.2683927708062;-1.8e-05 -9.53182893104904e-12 -11.9933808024341 -81.2729199440888;-1.7e-05 -9.53452598108609e-12 -11.9627407819086 -81.2774355666769;-1.6e-05 -9.53722167605435e-12 -11.9320990612107 -81.2819396379289;-1.5e-05 -9.53991601557073e-12 -11.9014556446956 -81.2864321572044;-1.4e-05 -9.54260899925228e-12 -11.8708105367181 -81.2909131238652;-1.3e-05 -9.54530062671627e-12 -11.8401637416337 -81.2953825372743;-1.2e-05 -9.54799089758017e-12 -11.809515263798 -81.2998403967965;-1.1e-05 -9.55067981146163e-12 -11.7788651075668 -81.3042867017982;-1e-05 -9.55336736797849e-12 -11.7482132772962 -81.3087214516476;-9e-06 -9.55605356674879e-12 -11.7175597773425 -81.3131446457143;-8e-06 -9.55873840739076e-12 -11.6869046120622 -81.3175562833698;-7e-06 -9.56142188952283e-12 -11.6562477858122 -81.321956363987;-6e-06 -9.56410401276361e-12 -11.6255893029493 -81.3263448869406;-5e-06 -9.56678477673192e-12 -11.594929167831 -81.3307218516069;-4e-06 -9.56946418104675e-12 -11.5642673848146 -81.3350872573637;-3e-06 -9.57214222532731e-12 -11.5336039582579 -81.3394411035908;-2e-06 -9.57481890919298e-12 -11.5029388925189 -81.3437833896693;-1e-06 -9.57749423226335e-12 -11.4722721919558 -81.348114114982]  x4=[-2.1e-05 5.01431529628906e-12 -11.7425908889822 -76.6919434564681;-2e-05 5.01581005508498e-12 -11.7136778736867 -76.696364859018;-1.9e-05 5.01730410102243e-12 -11.6847631936164 -76.700775361304;-1.8e-05 5.01879743388907e-12 -11.6558468528806 -76.7051749626992;-1.7e-05 5.02029005347267e-12 -11.626928855589 -76.7095636625785;-1.6e-05 5.02178195956109e-12 -11.5980092058516 -76.713941460318;-1.5e-05 5.02327315194231e-12 -11.5690879077784 -76.7183083552955;-1.4e-05 5.02476363040438e-12 -11.5401649654798 -76.7226643468905;-1.3e-05 5.02625339473547e-12 -11.5112403830664 -76.7270094344838;-1.2e-05 5.02774244472387e-12 -11.482314164649 -76.731343617458;-1.1e-05 5.02923078015793e-12 -11.4533863143387 -76.7356668951969;-1e-05 5.03071840082615e-12 -11.4244568362467 -76.7399792670863;-9e-06 5.03220530651708e-12 -11.3955257344847 -76.7442807325132;-8e-06 5.03369149701942e-12 -11.3665930131643 -76.7485712908663;-7e-06 5.03517697212193e-12 -11.3376586763975 -76.7528509415358;-6e-06 5.0366617316135e-12 -11.3087227282966 -76.7571196839134;-5e-06 5.03814577528311e-12 -11.279785172974 -76.7613775173925;-4e-06 5.03962910291985e-12 -11.2508460145424 -76.765624441368;-3e-06 5.0411117143129e-12 -11.2219052571147 -76.7698604552362;-2e-06 5.04259360925156e-12 -11.1929629048039 -76.7740855583952;-1e-06 5.0440747875252e-12 -11.1640189617235 -76.7782997502444]  x5=2.03919101606495e-05  V1=ones(3,3)  V2=ones(3,3)  I1=ones(3,3)  I2=ones(3,3)  nHarmo=1  Measurements=None
  Ground3 : powerlib/Elements/Ground  LConnTagsString=a
  "Grounding Transformer " : powerlib/Elements/Grounding Transformer   UNITS=pu  NominalPower="[100e6   60]"  NominalVoltage=25e3  ZeroSequenceImpedance_pu=[0.025 0.75]  MagnetizationBranch_pu=[500 500]  ZeroSequenceImpedance_SI=[0.052083 589.05]  MagnetizationBranch_SI=[1041.7 3.927e+005]  Measurements=None
  Conn1 : PMIOPort  Port=1  Side=Left
  Conn2 : PMIOPort  Port=2  Side=Left
  Conn3 : PMIOPort  Port=3  Side=Left
  connections:
  5-km Feeder/LConn1 -- Conn1/RConn1
  5-km Feeder/LConn2 -- Conn2/RConn1
  30-MW 2-Mvar Load/LConn1 -- 14-km Feeder/RConn1 -- 120 kV / 25 kV 47 MVA/RConn1 -- "Grounding Transformer "/LConn1
  30-MW 2-Mvar Load/LConn2 -- 14-km Feeder/RConn2 -- 120 kV / 25 kV 47 MVA/RConn2 -- "Grounding Transformer "/LConn2
  14-km Feeder/LConn2 -- 2-MW Load/LConn2 -- 5-km Feeder/RConn2
  30-MW 2-Mvar Load/LConn3 -- 14-km Feeder/RConn3 -- 120 kV / 25 kV 47 MVA/RConn3 -- "Grounding Transformer "/LConn3
  14-km Feeder/LConn1 -- 2-MW Load/LConn1 -- 5-km Feeder/RConn1
  "3.3ohms "/RConn1 -- Ground3/LConn1
  120 kV / 25 kV 47 MVA/LConn2 -- 120kV 2500MVA/RConn2
  "Grounding Transformer "/RConn1 -- "3.3ohms "/LConn1
  120 kV / 25 kV 47 MVA/LConn3 -- 120kV 2500MVA/RConn3
  Conn3/RConn1 -- 5-km Feeder/LConn3
  120 kV / 25 kV 47 MVA/LConn1 -- 120kV 2500MVA/RConn1
  14-km Feeder/LConn3 -- 2-MW Load/LConn3 -- 5-km Feeder/RConn3

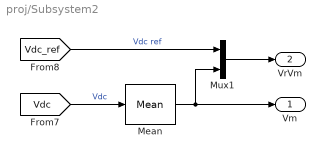
== system proj/Subsystem2 ==
  Mean : powerlib_meascontrol/Measurements/Mean  Freq=60  Vinit=0  Ts=1e-06
  Mux1 : Mux  Inputs=2
  Vm : Outport
  VrVm : Outport  Port=2
  wires:
  [Vdc_ref] -> Mux1/1  "Vdc ref"
  [Vdc] -> Mean/1  "Vdc"
  Mux1/1 -> VrVm/1
  Mean/1 -> Mux1/2, Vm/1

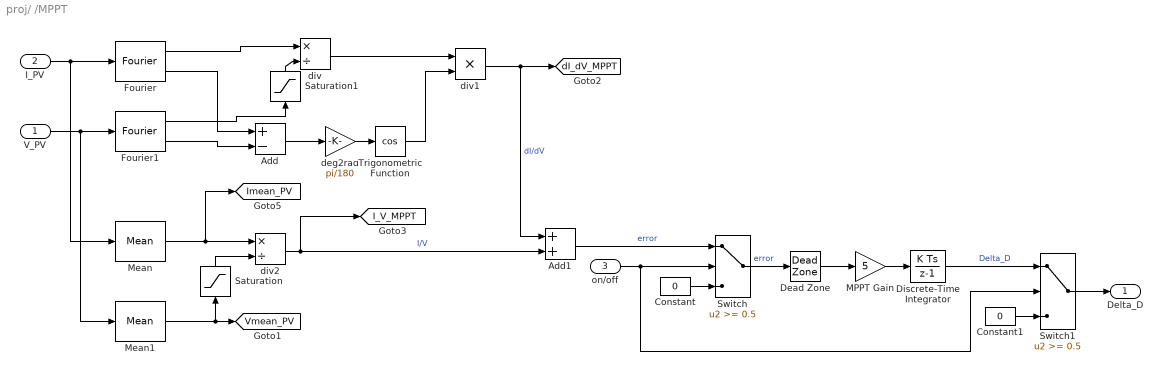
== system proj/ /MPPT ==
  V_PV : Inport
  I_PV : Inport  Port=2
  on/off : Inport  Port=3
  Add : Sum  Inputs=+-
  Add1 : Sum
  Constant : Constant  Value=0
  Constant1 : Constant  Value=0
  Dead Zone : DeadZone  LowerValue=-0.05  UpperValue=0.05  SaturateOnIntegerOverflow=on
  Discrete-Time Integrator : DiscreteIntegrator  SampleTime=1e-06  LimitOutput=on  UpperSaturationLimit=1  LowerSaturationLimit=-1
  Fourier : powerlib_meascontrol/Measurements/Fourier  Freq=1/T_MPPT  n=1  InInit=[0, 0]  Ts=1e-06
  Fourier1 : powerlib_meascontrol/Measurements/Fourier  Freq=1/T_MPPT  n=1  InInit=[0, 0]  Ts=1e-06
  MPPT Gain : Gain  Gain=5
  Mean : powerlib_meascontrol/Measurements/Mean  Freq=1/T_MPPT  Vinit=0  Ts=1e-06
  Mean1 : powerlib_meascontrol/Measurements/Mean  Freq=1/T_MPPT  Vinit=0  Ts=1e-06
  Saturation : Saturate  UpperLimit=inf  LowerLimit=eps
  Saturation1 : Saturate  UpperLimit=inf  LowerLimit=eps
  Switch : Switch  Threshold=0.5
  Switch1 : Switch  Threshold=0.5
  Trigonometric Function : Trigonometry  Operator=cos
  deg2rad : Gain  Gain=pi/180
  div : Product  Inputs=*/  RndMeth=Zero
  div1 : Product  Inputs=**  RndMeth=Zero
  div2 : Product  Inputs=*/  RndMeth=Zero
  Delta_D : Outport
  tag scope: I_V_MPPT=global, Imean_PV=global, Vmean_PV=global, dI_dV_MPPT=global
  wires:
  Dead Zone/1 -> MPPT Gain/1
  Switch/1 -> Dead Zone/1  "error"
  Saturation1/1 -> div/2
  Saturation/1 -> div2/2
  Switch1/1 -> Delta_D/1
  on/off/1 -> Switch/2, Switch1/2
  Constant1/1 -> Switch1/3
  Discrete-Time Integrator/1 -> Switch1/1  "Delta_D"
  Constant/1 -> Switch/3
  MPPT Gain/1 -> Discrete-Time Integrator/1
  Add1/1 -> Switch/1  "error"
  div2/1 -> Add1/2, [I_V_MPPT]  "I/V"
  Mean1/1 -> Saturation/1, [Vmean_PV]
  Mean/1 -> div2/1, [Imean_PV]
  div1/1 -> Add1/1, [dI_dV_MPPT]  "dI/dV"
  Trigonometric Function/1 -> div1/2
  div/1 -> div1/1
  deg2rad/1 -> Trigonometric Function/1
  Add/1 -> deg2rad/1
  Fourier1/1 -> Saturation1/1
  Fourier1/2 -> Add/2
  Fourier/2 -> Add/1
  V_PV/1 -> Mean1/1, Fourier1/1
  I_PV/1 -> Mean/1, Fourier/1
  Fourier/1 -> div/1
